simulink model "Problem_1_DVA"  (R2020b)
settings: Solver=VariableStepAuto  StartTime=0.0  StopTime=10.0  RelTol=1e-3
PreLoadFcn:
  | m1=50;
  | k1=50;
  | b=50;
  | k2=100;
  | m2=60;
settings Model: Creator=Manoj  LastModifiedBy=Windows 10

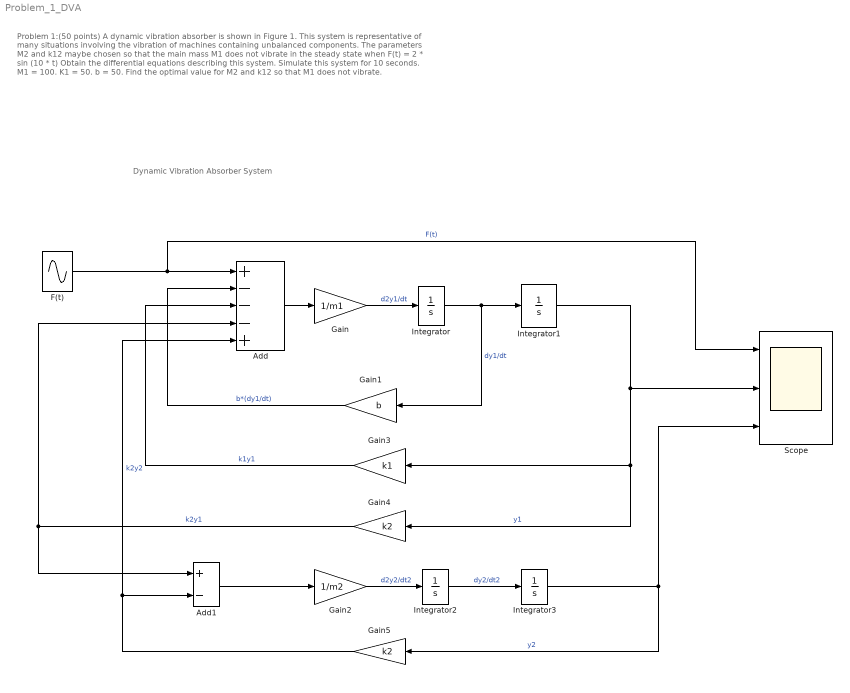
== system Problem_1_DVA ==
  note: Dynamic Vibration Absorber System
  note: Problem 1:(50 points) A dynamic vibration absorber is shown in Figure 1. This system is representative of many situations involving the vibration of machines containing unbalanced components. The parameters M2 and k12 maybe chosen so that the main mass M1 does not vibrate in the steady state when F(t) = 2 * sin (10 * t)
      | Obtain the differential equations describing this system.
      | Simulate this system for 10 seconds. M1 = 100. K1 = 50. b = 50.
      | Find the optimal value for M2 and k12 so that M1 does not vibrate.
  Add : Sum  Inputs=+---+
  Add1 : Sum  Inputs=+-
  F(t) : Sin  Amplitude=2  Frequency=10  SampleTime=0
  Gain : Gain  Gain=1/m1
  Gain1 : Gain  Gain=b
  Gain2 : Gain  Gain=1/m2
  Gain3 : Gain  Gain=k1
  Gain4 : Gain  Gain=k2
  Gain5 : Gain  Gain=k2
  Integrator{,1..3} (4 alike) : Integrator
  Scope : Scope  NumInputPorts=3
  wires:
  F(t)/1 -> Scope/1, Add/1  "F(t)"
  Gain/1 -> Integrator/1  "d2y1/dt"
  Gain1/1 -> Add/2  "b*(dy1/dt)"
  Add/1 -> Gain/1
  Integrator/1 -> Gain1/1, Integrator1/1  "dy1/dt"
  Integrator1/1 -> Gain4/1, Gain3/1, Scope/2  "y1"
  Gain3/1 -> Add/3  "k1y1"
  Gain4/1 -> Add/4, Add1/1  "k2y1"
  Add1/1 -> Gain2/1
  Gain2/1 -> Integrator2/1  "d2y2/dt2"
  Integrator2/1 -> Integrator3/1  "dy2/dt2"
  Integrator3/1 -> Gain5/1, Scope/3  "y2"
  Gain5/1 -> Add/5, Add1/2  "k2y2"
